simulink model "guzel"  (R2020a)
settings: Solver=VariableStepAuto  StartTime=0.0  StopTime=10.0  RelTol=1e-3
settings Model: Creator=muham  LastModifiedBy=muham

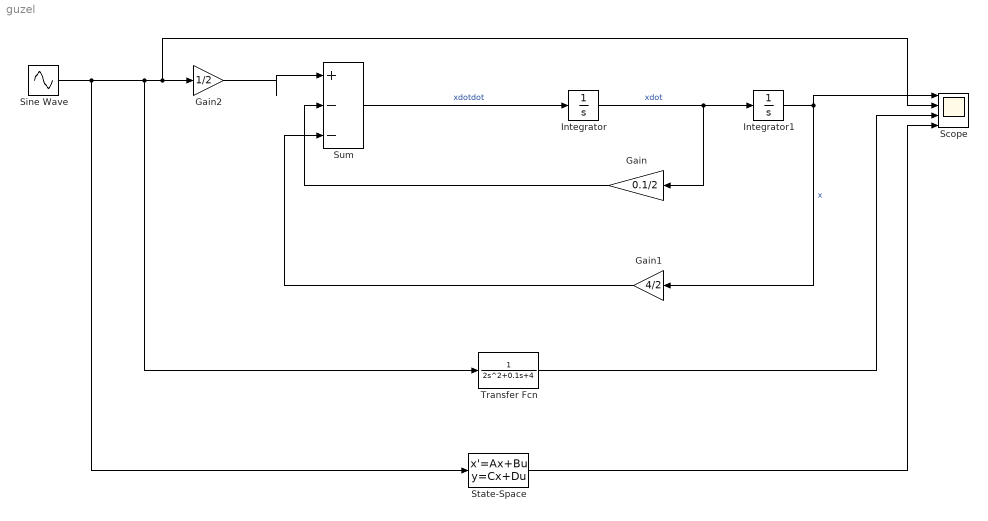
== system guzel ==
  Gain : Gain  Gain=0.1/2
  Gain1 : Gain  Gain=4/2
  Gain2 : Gain  Gain=1/2
  Integrator : Integrator
  Integrator1 : Integrator
  Scope : Scope  NumInputPorts=4
  Sine Wave : Sin  SampleTime=0
  State-Space : StateSpace  A=[0 1; -4/2 -0.1/2]  B=[0;1/2]  C=[1 0]  D=0  InitialCondition=0
  Sum : Sum  Inputs=|+--
  Transfer Fcn : TransferFcn  Denominator=[2 0.1 4]
  wires:
  Integrator/1 -> Gain/1, Integrator1/1  "xdot"
  Integrator1/1 -> Scope/1, Gain1/1  "x"
  Sum/1 -> Integrator/1  "xdotdot"
  Sine Wave/1 -> State-Space/1, Transfer Fcn/1, Scope/2, Gain2/1
  Gain2/1 -> Sum/1
  Gain/1 -> Sum/2
  Gain1/1 -> Sum/3
  Transfer Fcn/1 -> Scope/3
  State-Space/1 -> Scope/4
